simulink model "AM"  (R2022b)
settings: Solver=VariableStepAuto  StartTime=0.0  StopTime=2  RelTol=1e-3
settings Model: Creator=HP  LastModifiedBy=HP

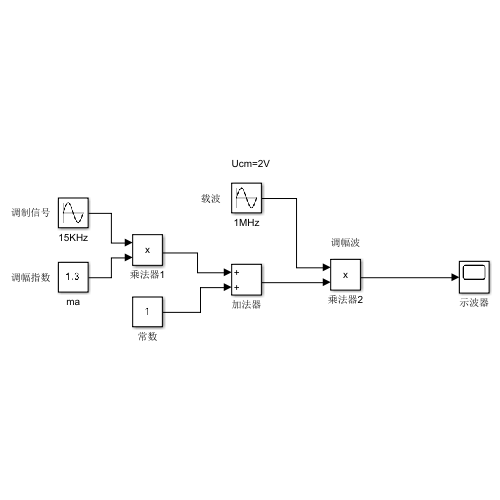
[thumbnail: Simulink's stored preview of the top-level diagram]
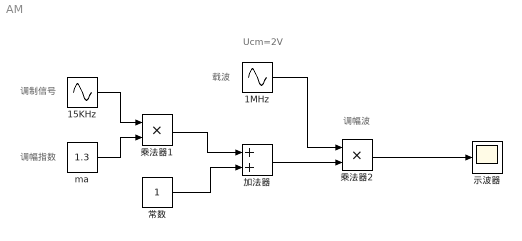
== system AM ==
  note: Ucm=2V
  note: 调幅波
  note: 调制信号
  note: 调幅指数
  note: 载波
  15KHz : Sin  Frequency=9.4248e+04  SampleTime=0
  1MHz : Sin  Amplitude=2  Frequency=6.2832e+06  SampleTime=0
  ma : Constant  Value=1.3
  乘法器1 : Product
  乘法器2 : Product
  加法器 : Sum
  常数 : Constant
  示波器 : Scope
  wires:
  常数/1 -> 加法器/2
  加法器/1 -> 乘法器2/2
  1MHz/1 -> 乘法器2/1
  乘法器2/1 -> 示波器/1
  乘法器1/1 -> 加法器/1
  15KHz/1 -> 乘法器1/1
  ma/1 -> 乘法器1/2
